simulink model "simulink_30_03"  (R2021a)
settings: Solver=FixedStepAuto  StartTime=0.0  StopTime=200  FixedStep=0.02  RelTol=1e-6
undefined symbols (not defined in the file): D_e, J_c, psi_sig, U_sig, V_sig
libraries: pid_lib x6, simulink x5, sharedutil x5, dspswit3 x1, aerolibutil x1
(part 2 of 3)

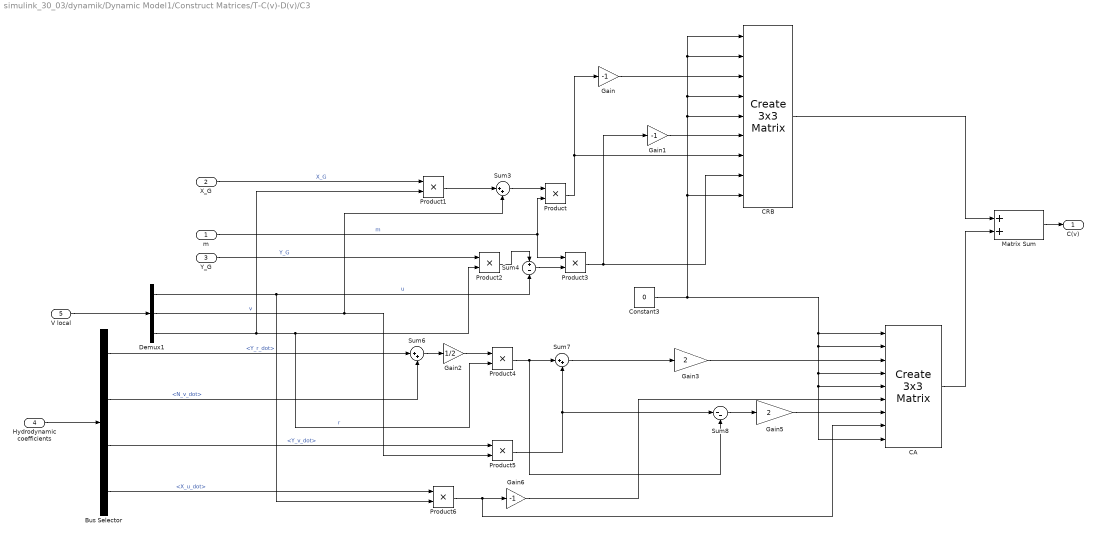
== system simulink_30_03/dynamik/Dynamic Model1/Construct Matrices/T-C(v)-D(v)/C3 ==
  m : Inport
  X_G : Inport  Port=2
  Y_G : Inport  Port=3
  Hydrodynamic coefficients : Inport  Port=4
  V local : Inport  Port=5
  " CRB" : sharedutil/Create 3x3 Matrix  aMode=aMode
      settings: SourceProductBaseCode=AE,PW,DR,MT,UV,VE
  Bus Selector : BusSelector  OutputSignals=Y_r_dot,N_v_dot,Y_v_dot,X_u_dot
  CA : sharedutil/Create 3x3 Matrix  aMode=aMode
      settings: SourceProductBaseCode=AE,PW,DR,MT,UV,VE
  Constant3 : Constant  Value=0
  Demux1 : Demux  Outputs=3
  Gain : Gain  Gain=-1
  Gain1 : Gain  Gain=-1
  Gain2 : Gain  Gain=1/2
  Gain3 : Gain  Gain=2
  Gain5 : Gain  Gain=2
  Gain6 : Gain  Gain=-1
  Matrix Sum : Sum
  Product{,1..6} (7 alike) : Product
  Sum3 : Sum  Inputs=|++
  Sum4 : Sum  Inputs=+-
  Sum6 : Sum  Inputs=|++
  Sum7 : Sum  Inputs=|++
  Sum8 : Sum  Inputs=|--
  C(v) : Outport  VectorParamsAs1DForOutWhenUnconnected=off
  wires:
  Bus Selector/1 -> Sum6/1  "<Y_r_dot>"
  Demux1/3 -> Product1/2, Product2/2, Product4/2  "r"
  Gain2/1 -> Product4/1
  CA/1 -> Matrix Sum/2
  Gain/1 -> " CRB"/3
  Bus Selector/2 -> Sum6/2  "<N_v_dot>"
  Sum3/1 -> Product/1
  Sum8/1 -> Gain5/1
  Product2/1 -> Sum4/1
  Sum6/1 -> Gain2/1
  Product5/1 -> Sum7/2, Sum8/1
  Gain1/1 -> " CRB"/6
  Product1/1 -> Sum3/1
  Y_G/1 -> Product2/1  "Y_G"
  Matrix Sum/1 -> C(v)/1
  Gain3/1 -> CA/3
  Gain6/1 -> CA/6
  Product6/1 -> Gain6/1, CA/8
  Demux1/2 -> Sum3/2, Product5/2  "v"
  Product4/1 -> Sum7/1, Sum8/2
  Product3/1 -> " CRB"/8, Gain1/1
  Gain5/1 -> CA/7
  " CRB"/1 -> Matrix Sum/1
  X_G/1 -> Product1/1  "X_G"
  Sum7/1 -> Gain3/1
  Product/1 -> " CRB"/7, Gain/1
  m/1 -> Product/2, Product3/1  "m"
  Constant3/1 -> " CRB"/5, " CRB"/4, " CRB"/2, " CRB"/1, " CRB"/9, CA/4, CA/5, CA/9, CA/2, CA/1
  Hydrodynamic coefficients/1 -> Bus Selector/1
  Bus Selector/4 -> Product6/1  "<X_u_dot>"
  Bus Selector/3 -> Product5/1  "<Y_v_dot>"
  Demux1/1 -> Sum4/2, Product6/2  "u"
  V local/1 -> Demux1/1
  Sum4/1 -> Product3/2

== system simulink_30_03/dynamik/Dynamic Model1/Construct Matrices/T-C(v)-D(v)/D ==
  Hydrodynamic Coefficients : Inport
  v_local : Inport  Port=2
  Bus Selector : BusSelector  OutputSignals=X_u,Y_v,Y_r,X_u|u|,Y_v|v|,Y_v|r|,Y_r|v|,N_v,N_r,Y_r|r|,N_v|v|,N_v|r|,N_r|r|,N_r|v|
  Demux1 : Demux  Outputs=3
  MATLAB Function : MATLAB Function  TreatAsAtomicUnit=on
  D_v : Outport
  wires:
  Hydrodynamic Coefficients/1 -> Bus Selector/1
  Demux1/3 -> MATLAB Function/3(r)
  MATLAB Function/1(D_v) -> D_v/1
  v_local/1 -> Demux1/1
  Bus Selector/1 -> MATLAB Function/4(X_u)  "<X_u>"
  Bus Selector/2 -> MATLAB Function/5(Y_v)  "<Y_v>"
  Bus Selector/14 -> MATLAB Function/16(N_r_abs_v)  "<N_r|v|>"
  Bus Selector/13 -> MATLAB Function/15(N_r_abs_r)  "<N_r|r|>"
  Bus Selector/12 -> ?  "<N_v|r|>"
  Bus Selector/11 -> MATLAB Function/14(N_v_abs_v)  "<N_v|v|>"
  Bus Selector/10 -> MATLAB Function/13(Y_r_abs_r)  "<Y_r|r|>"
  Bus Selector/9 -> MATLAB Function/7(N_r)  "<N_r>"
  Bus Selector/8 -> MATLAB Function/8(N_v)  "<N_v>"
  Bus Selector/7 -> MATLAB Function/12(Y_r_abs_v)  "<Y_r|v|>"
  Bus Selector/6 -> MATLAB Function/10(Y_v_abs_r)  "<Y_v|r|>"
  Bus Selector/5 -> MATLAB Function/9(Y_v_abs_v)  "<Y_v|v|>"
  Bus Selector/4 -> MATLAB Function/11(x_u_abs_u)  "<X_u|u|>"
  Bus Selector/3 -> MATLAB Function/6(Y_r)  "<Y_r>"
  Demux1/1 -> MATLAB Function/2(u)
  Demux1/2 -> MATLAB Function/1(v)

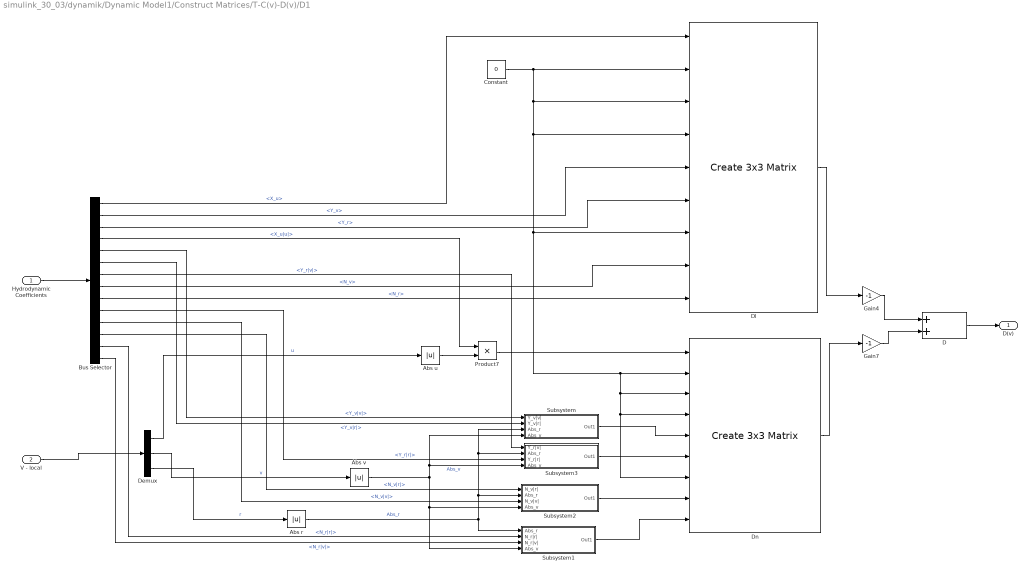
== system simulink_30_03/dynamik/Dynamic Model1/Construct Matrices/T-C(v)-D(v)/D1 ==
  Hydrodynamic Coefficients : Inport
  V - local : Inport  Port=2
  Abs r : Abs
  Abs u : Abs
  Abs v : Abs
  Bus Selector : BusSelector  OutputSignals=X_u,Y_v,Y_r,X_u|u|,Y_v|v|,Y_v|r|,Y_r|v|,N_v,N_r,Y_r|r|,N_v|v|,N_v|r|,N_r|r|,N_r|v|
  Constant : Constant  Value=0
  D : Sum
  Demux : Demux  Outputs=3
  Dl : sharedutil/Create 3x3 Matrix  aMode=aMode
      settings: SourceProductBaseCode=AE,PW,DR,MT,UV,VE
  Dn : sharedutil/Create 3x3 Matrix  aMode=aMode
      settings: SourceProductBaseCode=AE,PW,DR,MT,UV,VE
  Gain4 : Gain  Gain=-1
  Gain7 : Gain  Gain=-1
  Product7 : Product
  Subsystem : Subsystem
  Subsystem1 : Subsystem
  Subsystem2 : Subsystem
  Subsystem3 : Subsystem
  D(v) : Outport  VectorParamsAs1DForOutWhenUnconnected=off
  wires:
  Constant/1 -> Dn/7, Dn/4, Dn/3, Dn/2, Dl/7, Dl/4, Dl/3, Dl/2
  Abs u/1 -> Product7/2
  Abs r/1 -> Subsystem/3(Abs_r), Subsystem3/2("Abs_r "), Subsystem2/2(Abs_r), Subsystem1/1(Abs_r)  "Abs_r"
  Product7/1 -> Dn/1
  Abs v/1 -> Subsystem/4("Abs_v "), Subsystem3/4(Abs_v), Subsystem1/4(Abs_v), Subsystem2/4(Abs_v)  "Abs_v"
  Gain7/1 -> D/2
  Gain4/1 -> D/1
  Dl/1 -> Gain4/1
  Dn/1 -> Gain7/1
  D/1 -> D(v)/1
  Subsystem/1(Out1) -> Dn/5
  Subsystem1/1(Out1) -> Dn/9
  Subsystem2/1(Out1) -> Dn/8
  Subsystem3/1(Out1) -> Dn/6
  Hydrodynamic Coefficients/1 -> Bus Selector/1
  Bus Selector/5 -> Subsystem/1("Y_v|v| ")  "<Y_v|v|>"
  Bus Selector/6 -> Subsystem/2(Y_v|r|)  "<Y_v|r|>"
  Bus Selector/2 -> Dl/5  "<Y_v>"
  Bus Selector/7 -> Subsystem3/1(Y_r|v|)  "<Y_r|v|>"
  Bus Selector/10 -> Subsystem3/3(Y_r|r|)  "<Y_r|r|>"
  Bus Selector/11 -> Subsystem2/3(N_v|v|)  "<N_v|v|>"
  Bus Selector/8 -> Dl/8  "<N_v>"
  Bus Selector/12 -> Subsystem2/1(N_v|r|)  "<N_v|r|>"
  Bus Selector/14 -> Subsystem1/3(N_r|v|)  "<N_r|v|>"
  Bus Selector/9 -> Dl/9  "<N_r>"
  Bus Selector/13 -> Subsystem1/2(N_r|r|)  "<N_r|r|>"
  Bus Selector/1 -> Dl/1  "<X_u>"
  Bus Selector/4 -> Product7/1  "<X_u|u|>"
  Bus Selector/3 -> Dl/6  "<Y_r>"
  Demux/1 -> Abs u/1  "u"
  Demux/2 -> Abs v/1  "v"
  Demux/3 -> Abs r/1  "r"
  V - local/1 -> Demux/1

== system simulink_30_03/dynamik/Dynamic Model1/Construct Matrices/T-C(v)-D(v)/Tau ==
  F_1 : Inport
  F_2 : Inport  Port=2
  B1 : Inport  Port=3
  alpha_1 : Inport  Port=4
  alpha_2 : Inport  Port=5
  MATLAB Function : MATLAB Function  TreatAsAtomicUnit=on
  MATLAB Function1 : MATLAB Function  Commented=on  TreatAsAtomicUnit=on
  Out_T : Outport
  wires:
  F_1/1 -> MATLAB Function/1(F_1)
  MATLAB Function/1(y) -> Out_T/1
  B1/1 -> MATLAB Function/5(d)
  F_2/1 -> MATLAB Function/2(F_2)
  alpha_1/1 -> MATLAB Function/3(alpha_1)
  alpha_2/1 -> MATLAB Function/4(alpha_2)

== system simulink_30_03/dynamik/Dynamic Model1/Construct Matrices/T-C(v)-D(v)/Tau1 ==
  B : Inport
  Tstbd : Inport  Port=2
  Tport : Inport  Port=3
  Correction factor : Gain
  Mux : Mux  Inputs=3
  Product25 : Product
  Sum : Sum  Inputs=|++
  Sum1 : Sum  Inputs=|+-
  Ty : Constant  Value=0
  Tz : Gain  Gain=1/2
  T : Outport  VectorParamsAs1DForOutWhenUnconnected=off
  wires:
  Product25/1 -> Tz/1
  Tz/1 -> Mux/3  "Tz"
  Mux/1 -> T/1  "T"
  B/1 -> Product25/1  "B"
  Sum1/1 -> Product25/2
  Ty/1 -> Mux/2  "Ty"
  Tstbd/1 -> Correction factor/1  "Tstbd"
  Tport/1 -> Sum/1, Sum1/1  "Tport"
  Sum/1 -> Mux/1
  Correction factor/1 -> Sum/2, Sum1/2  "Tstbd"

== system simulink_30_03/dynamik/Dynamic Model1/Construct Matrices/T-C(v)-D(v)/D1/Subsystem ==
  "Y_v|v| " : Inport
  Y_v|r| : Inport  Port=2
  Abs_r : Inport  Port=3
  "Abs_v " : Inport  Port=4
  Product8 : Product
  Product9 : Product
  Sum10 : Sum  Inputs=|++
  Out1 : Outport  VectorParamsAs1DForOutWhenUnconnected=off
  wires:
  Y_v|r|/1 -> Product9/1
  Abs_r/1 -> Product9/2
  Product9/1 -> Sum10/2
  "Y_v|v| "/1 -> Product8/1
  Product8/1 -> Sum10/1
  "Abs_v "/1 -> Product8/2
  Sum10/1 -> Out1/1

== system simulink_30_03/dynamik/Dynamic Model1/Construct Matrices/T-C(v)-D(v)/D1/Subsystem1 ==
  Abs_r : Inport
  N_r|r| : Inport  Port=2
  N_r|v| : Inport  Port=3
  Abs_v : Inport  Port=4
  Product14 : Product
  Product15 : Product
  Sum13 : Sum  Inputs=|++
  Out1 : Outport  VectorParamsAs1DForOutWhenUnconnected=off
  wires:
  Product15/1 -> Sum13/1
  Sum13/1 -> Out1/1
  N_r|v|/1 -> Product14/1
  Product14/1 -> Sum13/2
  Abs_r/1 -> Product15/2
  N_r|r|/1 -> Product15/1
  Abs_v/1 -> Product14/2

== system simulink_30_03/dynamik/Dynamic Model1/Construct Matrices/T-C(v)-D(v)/D1/Subsystem2 ==
  N_v|r| : Inport
  Abs_r : Inport  Port=2
  N_v|v| : Inport  Port=3
  Abs_v : Inport  Port=4
  Product12 : Product
  Product13 : Product
  Sum12 : Sum  Inputs=|++
  Out1 : Outport  VectorParamsAs1DForOutWhenUnconnected=off
  wires:
  Sum12/1 -> Out1/1
  Product13/1 -> Sum12/1
  N_v|v|/1 -> Product12/1
  Product12/1 -> Sum12/2
  Abs_r/1 -> Product13/2
  Abs_v/1 -> Product12/2
  N_v|r|/1 -> Product13/1

== system simulink_30_03/dynamik/Dynamic Model1/Construct Matrices/T-C(v)-D(v)/D1/Subsystem3 ==
  Y_r|v| : Inport
  "Abs_r " : Inport  Port=2
  Y_r|r| : Inport  Port=3
  Abs_v : Inport  Port=4
  Product10 : Product
  Product11 : Product
  Sum11 : Sum  Inputs=|++
  Out1 : Outport  VectorParamsAs1DForOutWhenUnconnected=off
  wires:
  Product11/1 -> Sum11/2
  Product10/1 -> Sum11/1
  Sum11/1 -> Out1/1
  Y_r|v|/1 -> Product10/1
  "Abs_r "/1 -> Product11/2
  Y_r|r|/1 -> Product11/1
  Abs_v/1 -> Product10/2

== matlab function simulink_30_03/dynamik/Triggered Subsystem/MATLAB Function1 ==
  settings: updateMethod=DISCRETE
  data: u input; v input; w input; p input; q input; r input; x input; y input; z input; phi input; theta input; psi input; xdot output; n input; mp input; rp input; V_c input; beta_c input; F_1 input; F_2 input; alpha_1 input; alpha_2 input; U_tot output
function [xdot,U_tot] = otter(u, v, w, p, q, r, x, y, z, phi, theta, psi,n,mp,rp,V_c,beta_c,F_1,F_2,alpha_1,alpha_2)
% [xdot,U] = otter(x,n,mp,rp,V_c,beta_c) returns the speed U in m/s (optionally) 
% and the time derivative of the state vector: 
x = [u v w p q r x y z phi theta psi]'; 
% for the Maritime Robotics Otter USV, see www.maritimerobotics.com. 
% The length of the USV is L = 2.0 m, while the state vector is defined as:
%
%  u:     surge velocity          (m/s)
%  v:     sway velocity           (m/s)
%  w:     heave velocity          (m/s)
%  p:     roll velocity           (rad/s)
%  q:     pitch velocity          (rad/s)
%  r:     yaw velocity            (rad/s)
%  x:     position in x direction (m)
%  y:     position in y direction (m)
%  z:     position in z direction (m)
%  phi:   roll angle              (rad)
%  theta: pitch angle             (rad)
%  psi:   yaw angle               (rad)
%
% The other inputs are:
%
% n = [ n(1) n(2) ]' where
%    n(1): propeller shaft speed, left (rad/s)
%    n(2): propeller shaft speed, right (rad/s)
%
% mp = payload mass (kg), maximum 45 kg
%  rp = [xp, yp, zp]' (m) is the location of the payload w.r.t. the CO
%  V_c:     current speed (m/s)
%  beta_c:  current direction (rad)
%
% See, ExOtter.m and demoOtterUSVHeadingControl.slx
%
% Author:    Thor I. Fossen
% Date:      2019-07-17
% Revisions: 2021-04-25 added call to new function crossFlowDrag.m
%            2021-06-21 Munk moment in yaw is neglected
%            2021-07-22 Added a new state for the trim moment
%            2021-12-17 New method Xudot = -addedMassSurge(m,L,rho) 

% Check of input and state dimensions
if (length(x) ~= 12),error('x vector must have dimension 12!'); end
if (length(n) ~= 2),error('n vector must have dimension 2!'); end

% trim: theta = -7.5 deg corresponds to 13.5 cm less height aft maximum load
trim_setpoint = 280;

% trim_setpoint is a step input, which is filtered using the state trim_moment
persistent trim_moment;

if isempty(trim_moment)
   trim_moment = 0;
end

% % Main data
% g   = 9.81;         % acceleration of gravity (m/s^2)
% rho = 1025;         % density of water
% L = 2.0;            % length (m)
% B = 1.08;           % beam (m)
% m = 55.0;           % mass (kg)
% rg = [0.2 0 -0.2]'; % CG for hull only (m)
% R44 = 0.4 * B;      % radii of gyrations (m)
% R55 = 0.25 * L;
% R66 = 0.25 * L;
% T_yaw = 1;          % time constant in yaw (s)
% Umax = 6 * 0.5144;  % max forward speed (m/s)
% 
% % Data for one pontoon
% B_pont  = 0.25;     % beam of one pontoon (m)
% y_pont  = 0.395;    % distance from centerline to waterline area center (m)
% Cw_pont = 0.75;     % waterline area coefficient (-)
% Cb_pont = 0.4;      % block coefficient, computed from m = 55 kg


% Main data
g   = 9.81;         % acceleration of gravity (m/s^2)
rho = 1025;         % density of water
L = 6.969;          % length (m)
B = 3.465;          % beam (m)
m = 775;            % mass (kg)
rg = [0 0 -0.044]'; % CG for hull only (m)
% R44 = 0.4 * B;    % radii of gyrations (m)
% R55 = 0.25 * L;
% R66 = 0.25 * L;
R44 = 0.3171 * B; %0.78934 * B; %0.62879*B;  % radii of gyrations (m)
R55 = 0.18482 * L; %0.24044*L; 
R66 = 0.23465 * L; %0.38756*L; 
T_yaw = 1 ;%2.5;%1;          % time constant in yaw (s)
Umax = 8 * 0.5144;  % max forward speed (m/s)


% Data for one pontoon
B_pont  = 0.696;    % beam of one pontoon (m)
y_pont  = 1.3395;   % distance from centerline to waterline area center (m)
Cw_pont = 0.75;     % waterline area coefficient (-)
%Cb_pont = 0.4;      % block coefficient, computed from m = 55 kg
Cb_pont = 0.375; % overslagsberegning af Cb


%%%%%%%%%%%%%%%%%%%%%%%%%%%%%%%%%%%%%%%%%%%%%%%%%%%%%%%%%%%%%%%%%%%%%%%%%%

% State and current variables
nu = x(1:6);                                % velocities [u v w p q r]
nu1 = x(1:3);                               % velocities [u v w]
nu2 = x(4:6);                               % velocities [p q r]
eta = x(7:12);                              % positions [x y z phi theta psi ]
U = sqrt(nu(1)^2 + nu(2)^2 + nu(3)^2);      % speed
u_c = V_c * cos(beta_c - eta(6));           % current surge velocity
v_c = V_c * sin(beta_c - eta(6));           % current sway velocity
nu_r = nu - [u_c v_c 0 0 0 0]';             % relative velocity vector

% Inertia dyadic, volume displacement and draft
nabla = (m+mp)/rho;                         % volume
T = nabla / (2 * Cb_pont * B_pont*L);       % draft
Ig_CG = m * diag([R44^2, R55^2, R66^2]);    % only hull in CG
rg = (m*rg + mp*rp)/(m+mp);           % CG location corrected for payload
Ig = Ig_CG - m * Smtrx(rg)^2 - mp * Smtrx(rp)^2;  % hull + payload in CO

% Experimental propeller data including lever arms
l1 = -y_pont;                           % lever arm, left propeller (m)
l2 = y_pont;                            % lever arm, right propeller (m)
k_pos = 0.02216/2;                      % Positive Bollard, one propeller 
k_neg = 0.01289/2;                      % Negative Bollard, one propeller 
n_max = 300.42; %sqrt((0.5*24.4 * g)/k_pos);    % maximum propeller rev. (rad/s)
n_min = -300.42; %-sqrt((0.5*13.6 * g)/k_neg);    % minimum propeller rev. (rad/s)
F_max = 1000;
F_min = -1000;

% MRB and CRB (Fossen 2021)
I3 = eye(3);
O3 = zeros(3,3);

MRB_CG = [ (m+mp) * I3  O3
           O3           Ig ];
CRB_CG = [ (m+mp) * Smtrx(nu2)         O3
           O3               -Smtrx(Ig*nu2)  ];

H = Hmtrx(rg);              % Transform MRB and CRB from the CG to the CO 
MRB = H' * MRB_CG * H;
CRB = H' * CRB_CG * H;

% Hydrodynamic added mass (best practise)
Xudot = -addedMassSurge(m,L,rho);   
Yvdot = -1.5 * m;
Zwdot = -1.0 * m;
Kpdot = -0.2 * Ig(1,1);
Mqdot = -0.8 * Ig(2,2);
Nrdot = -1.7 * Ig(3,3);




MA = -diag([Xudot, Yvdot, Zwdot, Kpdot, Mqdot, Nrdot]);   
CA  = m2c(MA, nu_r);
CA(6,1) = 0; % Assume that the Munk moment in yaw can be neglected
CA(6,2) = 0; % These terms, if nonzero, must be balanced by adding nonlinear damping

% System mass and Coriolis-centripetal matrices
M = MRB + MA;
C = CRB + CA;

% Hydrostatic quantities (Fossen 2021)
Aw_pont = Cw_pont * L * B_pont;    % waterline area, one pontoon 
I_T = 2 * (1/12)*L*B_pont^3 * (6*Cw_pont^3/((1+Cw_pont)*(1+2*Cw_pont)))...
    + 2 * Aw_pont * y_pont^2;
I_L = 0.8 * 2 * (1/12) * B_pont * L^3;
KB = (1/3)*(5*T/2 - 0.5*nabla/(L*B_pont) );
BM_T = I_T/nabla;       % BM values
BM_L = I_L/nabla;
KM_T = KB + BM_T;       % KM values
KM_L = KB + BM_L;
KG = T - rg(3);
GM_T = KM_T - KG;       % GM values
GM_L = KM_L - KG;

G33 = rho * g * (2 * Aw_pont);      % spring stiffness
G44 = rho * g *nabla * GM_T;
G55 = rho * g *nabla * GM_L;

G_CF = diag([0 0 G33 G44 G55 0]);   % spring stiffness matrix in the CF
LCF = -0.2;
LCF = 0;
H = Hmtrx([LCF 0 0]);               % transform G_CF from the CF to the CO 
G = H' * G_CF * H;

% Natural frequencies
w3 = sqrt( G33/M(3,3) );         
w4 = sqrt( G44/M(4,4) );
w5 = sqrt( G55/M(5,5) );

% Linear damping terms (hydrodynamic derivatives)
    
if nu_r(1) < 1 && nu_r(1) > -1
%     if nu_r(1) < 0.5
%         Xu = -130;
%     else
    Xu = -130;
%    end
else 
     Xu = -51.3;
end

%Xu = -1.5 ;% -51.3;% -775; %(-24.4 * g / Umax);           % specified using the maximum speed  
Yv = -51.3;
Zw = -2 * 0.3 *w3 * M(3,3);      % specified using relative damping factors
Kp = -2 * 0.2 *w4 * M(4,4);
Mq = -2 * 0.4 *w5 * M(5,5);
Nr = -M(6,6) / T_yaw;            % specified using the time constant in T_yaw

% % Control forces and moments - with propeller revolution saturation 
% Thrust = zeros(2,1);
% for i = 1:1:2
%     if n(i) > n_max              % saturation, physical limits
%        n(i) = n_max; 
%     elseif n(i) < n_min
%        n(i) = n_min; 
%     end
%     
%    if n(i) > 0                          
%      Thrust(i) = k_pos * n(i)*abs(n(i));    % positive thrust (N) 
%    else
%      Thrust(i) = k_neg * n(i)*abs(n(i));    % negative thrust (N) 
%    end
% end
% 
% % Control forces and moments
% tau = [Thrust(1) + Thrust(2) 0 0 0 0 -l1 * Thrust(1) - l2 * Thrust(2) ]';

% Control forces and moments - with propeller revolution saturation 

if F_1 > F_max              % saturation, physical limits
  F_1 = F_max; 
elseif F_1 < F_min
  F_1 = F_min; 
end
if F_2 > F_max              % saturation, physical limits
  F_2 = F_max; 
elseif F_1 < F_min
  F_2 = F_min; 
end

% Control forces and moments
tau = [F_1*cos(alpha_1)+F_2*cos(alpha_2) F_1*sin(alpha_1)+F_2*sin(alpha_2) 0 0 0 F_1*y_pont*cos(alpha_1)-F_2*y_pont*cos(alpha_2)]';



% Linear damping using relative velocities + nonlinear yaw damping
Xh = Xu * nu_r(1);
Yh = Yv * nu_r(2); 
Zh = Zw * nu_r(3);
Kh = Kp * nu_r(4);
Mh = Mq * nu_r(5);
%Nh = Nr * (1 + 10 * abs(nu_r(6))) * nu_r(6);
Nh = Nr * (1 + 1 * abs(nu_r(6))) * nu_r(6);


tau_damp = [Xh Yh Zh Kh Mh Nh]';

% Strip theory: cross-flow drag integrals for Yh and Nh
tau_crossflow = crossFlowDrag(L,B_pont,T,nu_r);

% Ballast
g_0 = [0 0 0 0 trim_moment 0]';

% Kinematics
J = eulerang(eta(4),eta(5),eta(6));


%lig = tau + tau_damp + tau_crossflow - C * nu_r - G * eta - g_0   % til at
%finde forces

% Time derivative of the state vector - numerical integration; see ExOtter.m  
xdot = [ M \ ( tau + tau_damp + tau_crossflow - C * nu_r - G * eta - g_0)
         J * nu ];  
     
trim_moment = trim_moment + 0.05 * (trim_setpoint - trim_moment);
U_tot = U;
end

== matlab function simulink_30_03/MATLAB Function1 ==
  data: v input; y output
function y = fcn(v)
    if(v == 0.0)
        out = 0.00000000000000000001;
    
    else
        out = v;
    
    end
        

y = out;

== matlab function simulink_30_03/vel to thrust (Fx) ==
  data: u_con input; Fx output
function Fx = fcn(u_con)
    x_u = 51.3;
    x_uu = 72.4;
    %knob_2_ms = 0.5144;

    if (u_con < 0)
        k = -1;
    else
        k = 1;
    end
    
    
    
    
    if (u_con == 0)
        T = 0; 
    else
        T = 2 * (19.2 *abs(u_con)^2 + 1.5* abs(u_con) + 39)*k;
        %T = ((x_u + x_uu * abs(u)) * abs(u))*k;
    end

Fx = T;

== matlab function simulink_30_03/MATLAB Function2 ==
  data: tau input; y output; alpha input
function y = fcn(tau, alpha)
    if(alpha <= 1.   tau ==0)
        out = 0.0001;
    
    else
        out = v;
    
    end
        

y = out;

== matlab function simulink_30_03/vel to thrust (Fy) ==
  data: v input; Fy output
function Fy = fcn(v)

    x_u = 51.3;
    x_uu = 72.4 ;
    %knob_2_ms = 0.5144;
    k_side = 4; % factor for vel sideway

    
    if (v < 0)
        k = -1;
    else
        k = 1;
    end
    
    T = k_side*((x_u + x_uu * abs(v)) * abs(v))*k;

Fy = T;

== matlab function simulink_30_03/mixer/MATLAB Function ==
  data: F_x input; F_y input; tau input; F_1 output; d input; F_2 output; alpha1 output; alpha2 output
function [F_1, F_2, alpha1, alpha2] = fcn(F_x,F_y,tau,d)

    F1 = (0.5000*(F_x*tau + F_x^2*d - tau*(F_x - sqrt(F_x^2 + F_y^2)) - F_x*d*(F_x - sqrt(F_x^2 + F_y^2))))/(F_x*d);
    F2 = -(0.5000*(F_x*tau - F_x^2*d - tau*(F_x - sqrt(F_x^2 + F_y^2)) + F_x*d*(F_x - sqrt(F_x^2 + F_y^2))))/(F_x*d);
    alpha_1 = -2*atan((F_x - sqrt(F_x^2 + F_y^2))/F_y);
    alpha_2 = alpha_1;
    
    
    % sideway: alpha > 70 degrees
    if abs(alpha_1) >= 7*pi/18 && abs(alpha_1) <= 11*pi/18 || abs(alpha_1) <= 25*pi/18 && abs(alpha_1) >= 29*pi/18  
        
        % between +-180 degrees
        if alpha_1 > pi 
            alpha_1 = alpha_1 - 2 * pi;
        elseif alpha_1 < -pi
            alpha_1 = alpha_1 + 2 * pi;
        end       
        % determining the right angle and thrust    
        if alpha_1 > pi/2       %(above 90 degrees)
            alpha_1 = alpha_1 - pi;
        elseif alpha_1 < -pi/2  %(below -90 degrees)
            alpha_1 = alpha_1 + pi;
        end
        
%         fprintf("Er HER alpha 1 :---------")
%         disp(alpha_1)
        % if alpha is positvie 
        if alpha_1 >= 0 %&& alpha_1 < pi/2
            F1 = 1.4618*F_x + 1.0913*tau;
            F2 = (0.5000*F_x - 0.3733*tau - (1.3736*F_x*(2.0634e+18*F_x - 1.5405e+18*tau + 1.4142*sqrt(1.8196e+37*F_x^2 - 2.3394e+37*F_x*F_y + 2.0811e+37*F_x*tau + 8.5155e+36*F_y^2 - 1.7465e+37*F_y*tau + 1.0141e+37*tau^(2))))/(5.6687e+18*F_x - 4.1269e+18*F_y + 4.2320e+18*tau) + (F_y*(2.0634e+18*F_x - 1.5405e+18*tau + 1.4142*sqrt(1.8196e+37*F_x^2 - 2.3394e+37*F_x*F_y + 2.0811e+37*F_x*tau + 8.5155e+36*F_y^2 - 1.7465e+37*F_y*tau + 1.0141e+37*tau^(2))))/(5.6687e+18*F_x - 4.1269e+18*F_y + 4.2320e+18*tau) - (1.0255*tau*(2.0634e+18*F_x - 1.5405e+18*tau + 1.4142*sqrt(1.8196e+37*F_x^2 - 2.3394e+37*F_x*F_y + 2.0811e+37*F_x*tau + 8.5155e+36*F_y^2 - 1.7465e+37*F_y*tau + 1.0141e+37*tau^(2))))/(5.6687e+18*F_x - 4.1269e+18*F_y + 4.2320e+18*tau));
            alpha_1 = 7*pi/18; % 70 degrees
            alpha_2 = 2*atan((2.0634e+18*F_x - 1.5405e+18*tau + 1.4142*sqrt(1.8196e+37*F_x^2 - 2.3394e+37*F_x*F_y + 2.0811e+37*F_x*tau + 8.5155e+36*F_y^2 - 1.7465e+37*F_y*tau + 1.0141e+37*tau^(2)))/(5.6687e+18*F_x - 4.1269e+18*F_y + 4.2320e+18*tau));
%             fprintf("Er HER alpha positiv")
%             fprintf("F1 =")
%             disp(F1)
%             fprintf("F2 =")
%             disp(F2)    
%             fprintf("alpha1 =")
%             disp(alpha_1)
%             fprintf("alpah2 =")
%             disp(alpha_2) 
%             if alpha_2 < 0 && alpha_1 > 0
%                 alpha_2 = pi/2;
%                 F2 = -F2;
%             end
            
        else % if alpha is negative
            F1 = 1.4618*F_x + 1.0913*tau;
            F2 = 3.4268e-19*sqrt(1.8196e+37*F_x^2 + 2.3394e+37*F_x*F_y + 2.0811e+37*F_x*tau + 8.5155e+36*F_y^2 + 1.7465e+37*F_y*tau + 1.0141e+37*tau^(2));
            alpha_1 = -7*pi/18; % -70 degrees
            alpha_2 = 2*atan((1.5405e+18*tau - 2.0634e+18*F_x + 1.4142*sqrt(1.8196e+37*F_x^2 + 2.3394e+37*F_x*F_y + 2.0811e+37*F_x*tau + 8.5155e+36*F_y^2 + 1.7465e+37*F_y*tau + 1.0141e+37*tau^(2)))/(5.6687e+18*F_x + 4.1269e+18*F_y + 4.2320e+18*tau));
%             fprintf("Er HER alpha negativ")
%             fprintf("F1 =")
%             disp(F1)
%             fprintf("F2 =")
%             disp(F2)    
%             fprintf("alpha1 =")
%             disp(alpha_1)
%             fprintf("alpah2 =")
%             disp(alpha_2)        
        end
        
      
        % limitter for angle of pods of 88 degrees
                
        
%         % limmitter and angle determination
%         % angle alpha_2
%         % keeps angle between +-180 degrees
%         if alpha_2 > pi
%             alpha_2 = alpha_2 - 2 * pi;
%         elseif alpha_2 < -pi
%             alpha_2 = alpha_2 + 2 * pi;
%         end       
%         % determining the right angle and thrust    
%         if alpha_2 > pi/2 && alpha_2 < 11*pi/18      %(between 90 and 120 degrees)
%             alpha_2 = alpha_2 - pi;
%             F2 = (-1)*F2;
%         elseif alpha_2 < -pi/2 && alpha_2 > 11*pi/18 %(between -90 and -120 degrees)
%             alpha_2 = alpha_2 + pi;
%             F2 = (-1)*F2;
%         end
% 
%         % limitter for the thrusters for going sideway
%         if abs(F1) > T_max
%             %F1 = T_max;            
%             F1_old = F1;
%             F1 = T_max;
%             F2 = F1/(F1_old/F2);   
%         %elseif F1 < -T_max
%         %    F1 = -T_max;    
%         end
%         if abs(F2) > T_max
%             %F2 = T_max;
%             F2_old = F2;
%             F2 = T_max;
%             F1 = F2/(F2_old/F1);  
%         %elseif F2 < -T_max
%         %   F2 = -T_max;    
%         end
    end
  
     
    % makes shure that the thrusters are straith if no input in surge andsway direction 
    if F_x == F_y && F_x < 0.001 && F_x > -0.001
        alpha_1 = 0;
        alpha_2 = 0;
    end
        
    
    
F_1 = F1;
F_2 = F2;
alpha1 = alpha_1;
alpha2 = alpha_2;

== matlab function simulink_30_03/controllers/Trust1/MATLAB Function ==
  data: diff_psi input; T_stbd_u output; diff_v input; T_port_u output; T_stbd input; T_port input
function [T_stbd_u,T_port_u] = fcn(diff_psi,diff_v,T_stbd, T_port)

    T1_stbd = T_stbd+diff_v/2 + diff_psi;
    T1_port = T_port+diff_v/2 - diff_psi;  
  
    

T_stbd_u = T1_stbd;
T_port_u = T1_port;

== matlab function simulink_30_03/controllers/Trust1/MATLAB Function1 ==
  data: limit input; Tstbd output; T_port input; T_stbd input; Tport output
function [Tstbd,Tport] = fcn(limit, T_port, T_stbd)

    max_min = limit;

     
    T_stbd_out = T_stbd;
    T_port_out = T_port;
    
    
    if T_port_out < -max_min || T_stbd_out < -max_min
        
        T_port_diff = abs(T_port_out+max_min);
        T_stbd_diff = abs(T_stbd_out+max_min);
        
        if T_port_out < T_stbd_out && T_stbd_out <= 0
            T_port_out = -max_min;
            T_stbd_out = T_stbd_out + T_port_diff;
            
        elseif T_port_out < T_stbd_out && T_stbd_out > 0
            T_port_out = -max_min;
            T_stbd_out = T_stbd_out - T_port_diff; 
            
        elseif T_stbd_out < T_port_out && T_port_out <= 0
            T_stbd_out = -max_min;
            T_port_out = T_port_out + T_stbd_diff;
            
        elseif T_stbd_out < T_port_out && T_port_out > 0
            T_stbd_out = -max_min;
            T_port_out = T_port_out - T_stbd_diff;         
        end 
    end
  
    if T_port_out > max_min || T_stbd_out > max_min       
        T_port_diff = abs(T_port_out-max_min);
        T_stbd_diff = abs(T_stbd_out-max_min);
        
        if T_port_out > T_stbd_out && T_stbd_out <= 0
            T_port_out = max_min;
            T_stbd_out = T_stbd_out - T_port_diff;
            
        elseif T_port_out > T_stbd_out && T_stbd_out > 0
            T_port_out = max_min;
            T_stbd_out = T_stbd_out + T_port_diff; 
            
        elseif T_stbd_out > T_port_out && T_port_out <= 0
            T_stbd_out = max_min;
            T_port_out = T_port_out - T_stbd_diff;
            
        elseif T_stbd_out > T_port_out && T_port_out > 0
            T_stbd_out = max_min;
            T_port_out = T_port_out + T_stbd_diff;          
        end          
 
    end
    


Tstbd = T_stbd_out;
Tport = T_port_out;

== matlab function simulink_30_03/controllers/Trust1/Subsystem1/limit maks ==
  data: limit input; Tstbd output; T_port input; T_stbd input; Tport output
function [Tstbd,Tport] = fcn(limit, T_port, T_stbd)

    max_min = limit;

     
    T_stbd_out = T_stbd;
    T_port_out = T_port;
    
  
    if T_port_out > max_min || T_stbd_out > max_min       
        T_port_diff = abs(T_port_out-max_min);
        T_stbd_diff = abs(T_stbd_out-max_min);
        
        if T_port_out > T_stbd_out && T_stbd_out <= 0
            T_port_out = max_min;
            T_stbd_out = T_stbd_out - T_port_diff;
            
        elseif T_port_out > T_stbd_out && T_stbd_out > 0
            T_port_out = max_min;
            T_stbd_out = T_stbd_out + T_port_diff; 
            
        elseif T_stbd_out > T_port_out && T_port_out <= 0
            T_stbd_out = max_min;
            T_port_out = T_port_out - T_stbd_diff;
            
        elseif T_stbd_out > T_port_out && T_port_out > 0
            T_stbd_out = max_min;
            T_port_out = T_port_out + T_stbd_diff;          
        end          
 
    end
    


Tstbd = T_stbd_out;
Tport = T_port_out;

== matlab function simulink_30_03/controllers/Trust1/Subsystem1/limit min ==
  data: limit input; Tstbd output; T_port input; T_stbd input; Tport output
function [Tstbd,Tport] = fcn(limit, T_port, T_stbd)

    max_min = limit;

     
    T_stbd_ = T_stbd;
    T_port_ = T_port;
    
    
    if T_port < -max_min || T_stbd < -max_min
        
        T_port_diff = abs(T_port+max_min);
        T_stbd_diff = abs(T_stbd+max_min);
        
        if T_port < T_stbd && T_stbd <= 0
            T_port_ = -max_min;
            T_stbd_ = T_stbd + T_port_diff;
            
        elseif T_port < T_stbd && T_stbd > 0
            T_port_ = -max_min;
            T_stbd_ = T_stbd - T_port_diff; 
            
        elseif T_stbd < T_port && T_port <= 0
            T_stbd_ = -max_min;
            T_port_ = T_port + T_stbd_diff;
            
        elseif T_stbd < T_port && T_port > 0
            T_stbd_ = -max_min;
            T_port_ = T_port - T_stbd_diff;         
        end 
  
    end
    
    T_port_out = T_port_;
    T_stbd_out = T_stbd_;
    
Tport = T_port_out;
Tstbd = T_stbd_out;

== matlab function simulink_30_03/dynamik/Dynamic Model1/Construct Matrices/M/M-matrice ==
  data: m input; M_out output; x_g input; y_g input; I_z input; Xu_dot input; Yv_dot input; Yr_dot input; Nr_dot input; Nv_dot input
function M_out = fcn(m,x_g,y_g,I_z, Xu_dot, Yv_dot, Yr_dot, Nr_dot,Nv_dot)

%      M_RB = [m ,   0   , -m*y_g;
%              0 ,   m   ,  m*x_g;
%              -m*y_g , m*x_g ,    I_z];
%          
%      M_A = [-Xu_dot ,      0   ,    0   ;
%                0    ,  -Yv_dot , -Yr_dot;
%                0    ,  -Nv_dot , -Nr_dot];
%          
         

    M_RB = [m ,   0   ,    0;
            0 ,   m   ,  m*x_g;
            0 , m*x_g ,   I_z];


    M_A = [-Xu_dot ,      0   ,    0   ;
              0    ,  -Yv_dot , -Yr_dot;
              0    ,  -Yr_dot , -Nr_dot];
   



    M = M_A + M_RB;

    m_inv = inv(M);


M_out = M;

== matlab function simulink_30_03/dynamik/Dynamic Model1/Construct Matrices/T-C(v)-D(v)/C1/MATLAB Function ==
  data: v input; u input; r input; y output; m input; x_g input; Xu_dot input; Yv_dot input; Yr_dot input
function y = fcn(v, u,r, m,x_g, Xu_dot, Yv_dot, Yr_dot)

    
    C_RB = [    0       ,     0     , -m*(x_g*r+v);
                0       ,     0     ,      m*u    ;
            m*(x_g*r+v) ,   -m*u    ,       0     ]



    C_A = [           0      ,     0     , Yv_dot*v+Yr_dot*r;
                      0      ,     0     ,     -Xu_dot*u    ;
            -Yv_dot*v-Yr_dot ,  Xu_dot*u ,         0        ]


    C = C_A + C_RB









y = C;

== matlab function simulink_30_03/dynamik/Dynamic Model1/Construct Matrices/T-C(v)-D(v)/C2/MATLAB Function ==
  data: v input; u input; r input; y output; m input; x_g input; Xu_dot input; Yv_dot input; Yr_dot input
function y = fcn(v, u,r, m,x_g, Xu_dot, Yv_dot, Yr_dot)

    
    C_RB = [    0       ,     0     , -m*(x_g*r+v);
                0       ,     0     ,      m*u    ;
            m*(x_g*r+v) ,   -m*u    ,       0     ]



    C_A = [           0      ,     0     , Yv_dot*v+Yr_dot*r;
                      0      ,     0     ,     -Xu_dot*u    ;
            -Yv_dot*v-Yr_dot ,  Xu_dot*u ,         0        ]


    C = C_A + C_RB









y = C;

== matlab function simulink_30_03/dynamik/Dynamic Model1/Construct Matrices/T-C(v)-D(v)/D/MATLAB Function ==
  data: v input; u input; r input; X_u input; D_v output; Y_v input; Y_r input; N_r input; N_v input; Y_v_abs_v input; Y_v_abs_r input; x_u_abs_u input; Y_r_abs_v input; Y_r_abs_r input; N_v_abs_v input; N_r_abs_r input; N_r_abs_v input
function D_v = fcn(v,u,r, X_u, Y_v, Y_r, N_r, N_v, Y_v_abs_v, Y_v_abs_r, x_u_abs_u, Y_r_abs_v, Y_r_abs_r, N_v_abs_v, N_r_abs_r, N_r_abs_v)
    %v = v_(1);
    %u = v_(2);
    %r = v_(3);


    D_RB = [-X_u ,   0  ,  0 ;
              0  , -Y_v , -Y_r;
             0   , -N_v , -N_r];
                
                  
    D_A = [-(x_u_abs_u)*abs(u)   ,                 0                          ,                         0                 ;
                      0          , -(Y_v_abs_v)*(abs(v))+(Y_v_abs_r)*(abs(r)) , -((Y_r_abs_v)*(abs(v))+(Y_r_abs_r)*(abs(r)));
                      0          , -(N_v_abs_v)*(abs(v))+(Y_v_abs_r)*(abs(r)) , -((N_r_abs_v)*(abs(v))+(N_r_abs_r)*(abs(r)))];
        
        

    D = D_RB + D_A;


D_v = D;

== matlab function simulink_30_03/dynamik/Dynamic Model1/Construct Matrices/T-C(v)-D(v)/Tau/MATLAB Function ==
  data: F_1 input; y output; F_2 input; alpha_1 input; alpha_2 input; d input
function y = fcn(F_1, F_2, alpha_1, alpha_2, d)
  
    % tau = [tau_x ; tau_y ; tau_z];
% 
%     force = [  F_1*cos(alpha_1)+F_2*cos(alpha_2)   ;
%                F_1*sin(alpha_1)+F_2*sin(alpha_2)   ;
%              F_1*d*cos(alpha_1)-F_2*d*cos(alpha_2)];
    
    force = [  F_1*cos(alpha_1)+F_2*cos(alpha_2)   ;
               F_1*sin(alpha_1)+F_2*sin(alpha_2)   ;
             F_1*d*cos(alpha_1)-F_2*d*cos(alpha_2)];     
    
y = force;

== matlab function simulink_30_03/dynamik/Dynamic Model1/Construct Matrices/T-C(v)-D(v)/Tau/MATLAB Function1 ==
  data: T_stbd input; y output; T_port input; B input
function y = fcn(T_stbd, T_port, B)
  
    % tau = [tau_x ; tau_y ; tau_z];

    tau = [   T_port + T_stbd   ;
                     0          ;
           (B*(T_port-T_stbd)/2)];
y = tau;

== matlab function simulink_30_03/limmitter and angle//thrust  ==
  data: F_1 input; F1 output; F_2 input; F2 output; alpha_in_1 input; alpha1 output; alpha_in_2 input; alpha2 output
function [F1, F2, alpha1, alpha2] = fcn(F_1,F_2, alpha_in_1, alpha_in_2)
%    fprintf("input_______input_")
%    fprintf("alpha_______input_ = ")
%    disp(alpha_in_1)
%    fprintf("F1_______input_ = ")
%    disp(F_1)  
%    
   
   
    T_max = 1000; % max for trust in both positiv and negativ direction 

  
    %if abs(alpha_in_1) < 7*pi/18 && abs(alpha_in_1) >= 0 
    % sway manuvering (abs(alpha > 70 degrees)) 
    if abs(alpha_in_1) >= 7*pi/18 && abs(alpha_in_1) <= 11*pi/18 || abs(alpha_in_1) <= 25*pi/18 && abs(alpha_in_1) >= 29*pi/18  % manuvering up to 
        
        % limmitter and angle determination
        % angle alpha_2
        % keeps angle between +-180 degrees
        if alpha_in_2 > pi
            alpha_in_2 = alpha_in_2 - 2 * pi;
        elseif alpha_in_2 < -pi
            alpha_in_2 = alpha_in_2 + 2 * pi;
        end       
        % determining the right angle and thrust    
        if alpha_in_2 > pi/2 && alpha_in_2 <= 11*pi/18      %(between 90 and 160 degrees)
            alpha_in_2 = alpha_in_2 - pi;
            F_2 = (-1)*F_2;
        elseif alpha_in_2 < -pi/2 && alpha_in_2 >= -11*pi/18 %(between -90 and -160 degrees)
            alpha_in_2 = alpha_in_2 + pi;
            F_2 = (-1)*F_2;
        end
        


        % limitter for the thrusters for going sideway
        if abs(F_1) > T_max
            if F_1 < 0
               T_max = (-1)*T_max; 
            end
            %F1 = T_max;            
            F1_old = F_1;
            F_1 = T_max;
            F_2 = F_1/(F1_old/F_2);   
        %elseif F1 < -T_max
        %    F1 = -T_max;    
        end
        if abs(F_2) > T_max
            if F_2 < 0
               T_max = (-1)*T_max; 
            end
            %F2 = T_max;
            F2_old = F_2;
            F_2 = T_max;
            F_1 = F_2/(F2_old/F_1);  
        %elseif F2 < -T_max
        %   F2 = -T_max;    
        end
  
        
        %pod angle limitter (88 degrees)
        if alpha_in_2 >= 22*pi/45 
            alpha_in_2 = 22*pi/45;
        elseif alpha_in_2 <= -22*pi/45 
            alpha_in_2 = -22*pi/45;
        end
        
        % solution for going straight in y direction
        if alpha_in_1 == 7*pi/18 && alpha_in_2 < 0
           alpha_in_2 = -alpha_in_2;
           F_2 = -F_2;
        end
        
 
        % returning results
        F_1_out = F_1;           
        F_2_out = F_2;
        alpha_out_1 = alpha_in_1;
        alpha_out_2 = alpha_in_2;
        
        
        
        
        
    else % manuuvering alpha less than 70 degrees     
        
        % if F1 is larger than the limit and F2 is positive
        if (F_1 > T_max && abs(F_2) < abs(F_1))
            diff = F_1 - T_max;  

            % if diff is out of range and F_1 > 0
            if ((abs(diff) > T_max)&& ((F_2 > 0) && (((F_2 - diff) > T_max) || (F_2 - diff) < -T_max)) ||  (F_2 < 0) && (((F_2 + diff) > T_max) || (F_2 + diff) < -T_max))             
                F_1_old = F_1;
                F_1 = T_max;
                F_2 = F_1/(F_1_old/F_2);
%                 fprintf("Er HER 1_special")

            elseif (F_2 >= 0)      %F2 is positive
                F_1 = F_1 - diff;
                F_2 = F_2 - diff;
%                 fprintf("Er HER 1_1")
            else                   %F2 is negative
                F_1 = F_1 - diff;
                F_2 = F_2 + diff; 
%                 fprintf("Er HER 1_2")
            end
        end    

        % if F2 is larger than the limit        
        if (F_2 > T_max && abs(F_2) > abs(F_1))          
            diff = F_2 - T_max;  

            % if diff is out of range and F_2 > 0
            if ((abs(diff) > T_max)&& ((F_1 > 0) && (((F_1 - diff) > T_max) || (F_1 - diff) < -T_max)) ||  (F_1 < 0) && (((F_1 + diff) > T_max) || (F_1 + diff) < -T_max))  
                F_2_old = F_2;
                F_2 = T_max;
                F_1 = F_2/(F_2_old/F_1);
%                 fprintf("Er HER 2_special")  

            elseif (F_1 >= 0)      %F1 is positive
                F_1 = F_1 - diff;
                F_2 = F_2 - diff;
%                 fprintf("Er HER 2_1")
            else                   %F1 is negative
                F_1 = F_1 + diff;
                F_2 = F_2 - diff; 
%                 fprintf("Er HER 2_2")
            end
        end

        % if F1 is below the limit
        if (F_1 < -T_max && abs(F_2) < abs(F_1))
            diff = F_1 - (-T_max); 

            % if diff is out of range and F_1 < 0
            if ((abs(diff) > T_max) && ((F_2 > 0) && (((F_2 + diff) > T_max) || (F_2 + diff) < -T_max)) ||  (F_2 < 0) && (((F_2 - diff) > T_max) || (F_2 - diff) < -T_max))  
                F_1_old = F_1;
                F_1 = -T_max;
                F_2 = F_1/(F_1_old/F_2);
%                 fprintf("Er HER 3_special")

            elseif (F_2 >= 0)      %F2 is positive
                F_1 = F_1 - diff;
                F_2 = F_2 + diff;
%                 fprintf("Er HER 3_1")
            else                   %F2 is negattive
                F_1 = F_1 - diff;
                F_2 = F_2 - diff;
%                 fprintf("Er HER 3_2")
            end
        end

        % if F2 is below the limit
        if (F_2 < -T_max && abs(F_2) > abs(F_1))
            diff = F_2 - (-T_max);

            % if diff is out of range and F_2 < 0
            if ((abs(diff) > T_max) && ((F_1 > 0) && (((F_1 - diff) > T_max) || (F_1 - diff) < -T_max)) ||  (F_1 < 0) && (((F_1 + diff) > T_max) || (F_2 + diff) < -T_max))  
                F_2_old = F_2;
                F_2 = -T_max;
                F_1 = F_2/(F_2_old/F_1);
%                 fprintf("Er HER 4_special")

            elseif (F_1 >= 0)     %F1 is positive
                F_1 = F_1 + diff;
                F_2 = F_2 - diff;
%                 fprintf("Er HER 4_1")
            else                  %F1 is negative
                F_1 = F_1 - diff;
                F_2 = F_2 - diff;    
%                 fprintf("Er HER 4_2")
            end
        end



        % angle alfa 
        % between +-180 degrees
        if alpha_in_1 > pi 
            alpha_in_1 = alpha_in_1 - 2 * pi;
        elseif alpha_in_1 < -pi 
            alpha_in_1 = alpha_in_1 + 2 * pi;
        end      
        fprintf("alpha = ")
        disp(alpha_in_1)
        fprintf("F1 = ")
        disp(F_1)
        % determining the right angle and thrust    
        if alpha_in_1 > pi/2       %(above 90 degrees)
            alpha_out = alpha_in_1 - pi;
            F_1_out = (-1)*F_1;
            F_2_out = (-1)*F_2;
%             fprintf("1-------- alpha>pi/2 ---------")
        elseif alpha_in_1 < -pi/2  %(below -90 degrees)
            alpha_out = alpha_in_1 + pi;
            F_1_out = (-1)*F_1;
            F_2_out = (-1)*F_2;
%             %fprintf("2-------- alpha<pi/2 ---------")
            
%         if alpha_in_1 > pi/2
%             alpha_out = alpha_in_1 - (2*pi);
%             F_1_out = (-1)*F_1;
%             F_2_out = (-1)*F_2;
% 
%         elseif alpha_in_1 < -pi/2
%             alpha_out = alpha_in_1 + 180;
%             F_1_out = (-1)*F_1;
%             F_2_out = (-1)*F_2;

        else 
            alpha_out = alpha_in_1;
            F_1_out = F_1;
            F_2_out = F_2;
        end
       
        alpha_out_1 = alpha_out;
        alpha_out_2 = alpha_out_1;
     
    end

  

      
F1 = F_1_out;
F2 = F_2_out;
alpha1 = alpha_out_1;
alpha2 = alpha_out_2;

== matlab function simulink_30_03/MATLAB Function3 ==
  data: alpha_in input; alpha output; F_1_in input; F_2_in input; F_1 output; F_2 output
function [alpha,F_1,F_2] = fcn(alpha_in, F_1_in, F_2_in)
    
    if alpha_in > pi/2
        alpha_out = alpha_in - (2*pi);
        F_1_out = (-1)*F_1_in;
        F_2_out = (-1)*F_2_in;
     
    elseif alpha_in < -pi/2
        alpha_out = alpha_in + 180;
        F_1_out = (-1)*F_1_in;
        F_2_out = (-1)*F_2_in;
  
    else 
        alpha_out = alpha_in;
        F_1_out = F_1_in;
        F_2_out = F_2_in;
    end


    
    
 
    
    

alpha = alpha_out;
F_1 = F_1_out;
F_2 = F_2_out;

== matlab function simulink_30_03/Subsystem/MATLAB Function ==
  data: F_x input; F_1 output; F_y input; tau input; d input; F_2 output; alpha1 output
function [F_1, F_2, alpha1] = fcn(F_x,F_y,tau,d)
    
    alpha_1 = 1.2217; % 70 degrees
    F1 = 1.4618*F_x + 1.0913 * tau;
    F2 = 0.5000*F_x - 0.3733*tau - (1.3736*F_x*(2.0634e+18*F_x - 1.5405e+18*tau + 1.4142*sqrt(1.8196e+37*F_x^2 - 2.3394e+37*F_x*F_y + 2.0811e+37*F_x*tau + 8.5155e+36*F_y^2 - 1.7465e+37*F_y*tau + 1.0141e+37*tau^sym(2))))/(5.6687e+18*F_x - 4.1269e+18*F_y + 4.2320e+18*tau) + (F_y*(2.0634e+18*F_x - 1.5405e+18*tau + 1.4142*sqrt(1.8196e+37*F_x^2 - 2.3394e+37*F_x*F_y + 2.0811e+37*F_x*tau + 8.5155e+36*F_y^2 - 1.7465e+37*F_y*tau + 1.0141e+37*tau^sym(2))))/(5.6687e+18*F_x - 4.1269e+18*F_y + 4.2320e+18*tau) - (1.0255*tau*(2.0634e+18*F_x - 1.5405e+18*tau + 1.4142*sqrt(1.8196e+37*F_x^2 - 2.3394e+37*F_x*F_y + 2.0811e+37*F_x*tau + 8.5155e+36*F_y^2 - 1.7465e+37*F_y*tau + 1.0141e+37*tau^sym(2))))/(5.6687e+18*F_x - 4.1269e+18*F_y + 4.2320e+18*tau);
    alpha_2 = 2*atan((2.0634e+18*F_x - 1.5405e+18*tau + 1.4142*sqrt(1.8196e+37*F_x^2 - 2.3394e+37*F_x*F_y + 2.0811e+37*F_x*tau + 8.5155e+36*F_y^2 - 1.7465e+37*F_y*tau + 1.0141e+37*tau^sym(2)))/(5.6687e+18*F_x - 4.1269e+18*F_y + 4.2320e+18*tau));
    
    if F_x == F_y && F_x < 0.001 && F_x > -0.001
        alpha_1 = 0;
    end
    
F_1 = F1;
F_2 = F2;
alpha1 = alpha_1;
alpha2 = alpha_2

== matlab function simulink_30_03/MATLAB Function ==
  data: u input; y output
function y = fcn(u)
    if(u == 0.0)
        out = 0.00000000000000000001;
    
    else
        out = u;
    
    end
        

y = out;
